simulink model "LQR"  (R2025b)
settings: Solver=VariableStepAuto  StartTime=0.0  StopTime=10.0  RelTol=1e-3
undefined symbols (not defined in the file): A, B, K_LQR_i, K_LQR_x, n, X0, x_ref
settings Model: Creator=salvo  LastModifiedBy=salvo

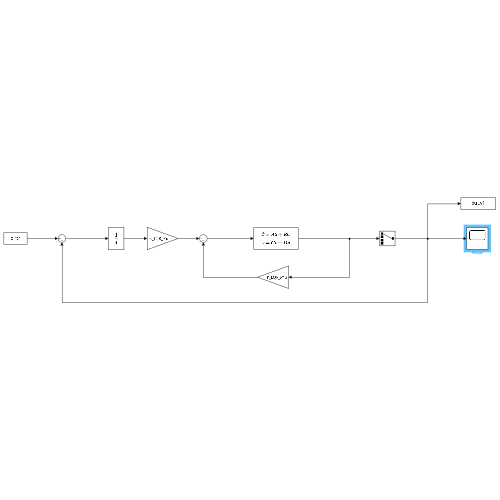
[thumbnail: Simulink's stored preview of the top-level diagram]
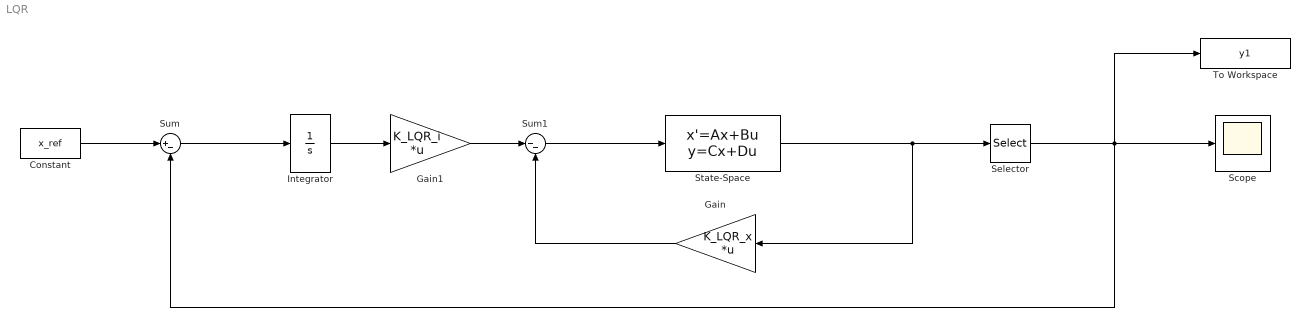
== system LQR ==
  Constant : Constant  Value=x_ref
  Gain : Gain  Gain=K_LQR_x  Multiplication=Matrix(K*u)
  Gain1 : Gain  Gain=K_LQR_i  Multiplication=Matrix(K*u)
  Integrator : Integrator
  Scope : Scope
      settings: ActiveDisplayYMinimum=0.038673610957029772  ActiveDisplayYMaximum=0.21794039197707538
  Selector : Selector  InputPortWidth=4  IndexOptions=Index vector (dialog)  Indices=[1]  OutputSizes=1
  State-Space : StateSpace  A=A  B=B  C=eye(n)  D=zeros(n,1)  InitialCondition=X0
  Sum : Sum  Inputs=|+-
  Sum1 : Sum  Inputs=|--
  To Workspace : ToWorkspace  VariableName=y1  SaveFormat=Timeseries  SampleTime=-1
  wires:
  Gain1/1 -> Sum1/1
  Sum1/1 -> State-Space/1
  Gain/1 -> Sum1/2
  State-Space/1 -> Selector/1, Gain/1
  Integrator/1 -> Gain1/1
  Constant/1 -> Sum/1
  Sum/1 -> Integrator/1
  Selector/1 -> To Workspace/1, Scope/1, Sum/2
